simulink model "SanityCheckY"  (R2023a)
settings: Solver=VariableStepAuto  StartTime=0.0  StopTime=10.0  RelTol=1e-3
settings Model: Creator=aan18022  LastModifiedBy=aan18022

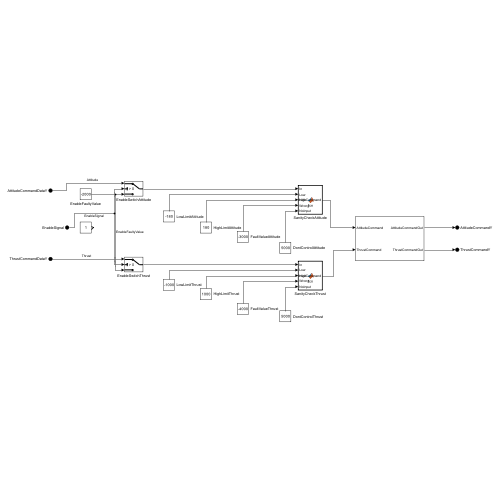
[thumbnail: Simulink's stored preview of the top-level diagram]
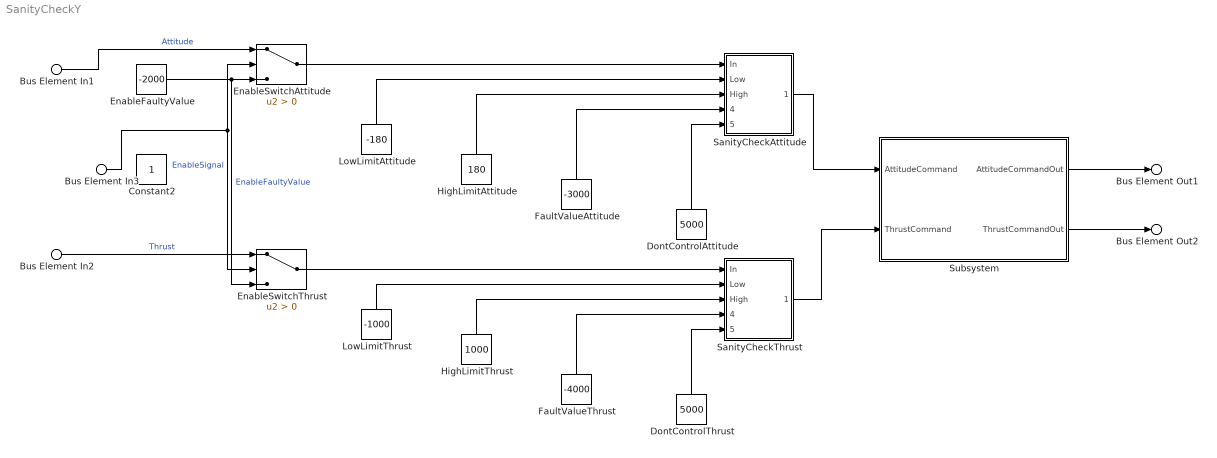
== system SanityCheckY ==
  Bus Element In3 : Inport  PortName=EnableSignal
  Bus Element In1 : Inport  Port=2  PortName=AttitudeCommandDataY
  Bus Element In2 : Inport  Port=3  PortName=ThrustCommandDataY
  Constant2 : Constant
  DontControlAttitude : Constant  Value=5000
  DontControlThrust : Constant  Value=5000
  EnableFaultyValue : Constant  Value=-2000
  EnableSwitchAttitude : Switch  Criteria=u2 > Threshold  SaturateOnIntegerOverflow=off  InputSameDT=off
  EnableSwitchThrust : Switch  Criteria=u2 > Threshold  SaturateOnIntegerOverflow=off  InputSameDT=off
  FaultValueAttitude : Constant  Value=-3000
  FaultValueThrust : Constant  Value=-4000
  HighLimitAttitude : Constant  Value=180
  HighLimitThrust : Constant  Value=1000
  LowLimitAttitude : Constant  Value=-180
  LowLimitThrust : Constant  Value=-1000
  SanityCheckAttitude : MATLAB Function  TreatAsAtomicUnit=on
  SanityCheckThrust : MATLAB Function  TreatAsAtomicUnit=on
  Subsystem : Subsystem
  Bus Element Out1 : Outport  PortName=AttitudeCommandY
  Bus Element Out2 : Outport  Port=2  PortName=ThrustCommandY
  wires:
  DontControlThrust/1 -> SanityCheckThrust/5(NoInput)
  HighLimitAttitude/1 -> SanityCheckAttitude/3(High)
  DontControlAttitude/1 -> SanityCheckAttitude/5(NoInput)
  EnableFaultyValue/1 -> EnableSwitchAttitude/3, EnableSwitchThrust/3  "EnableFaultyValue"
  Bus Element In3/1 -> EnableSwitchThrust/2, EnableSwitchAttitude/2  "EnableSignal"
  EnableSwitchThrust/1 -> SanityCheckThrust/1(In)
  FaultValueThrust/1 -> SanityCheckThrust/4(Wrong)
  HighLimitThrust/1 -> SanityCheckThrust/3(High)
  LowLimitThrust/1 -> SanityCheckThrust/2(Low)
  SanityCheckAttitude/1(AttitudeCommand) -> Subsystem/1(AttitudeCommand)
  Bus Element In2/1 -> EnableSwitchThrust/1  "Thrust"
  LowLimitAttitude/1 -> SanityCheckAttitude/2(Low)
  Bus Element In1/1 -> EnableSwitchAttitude/1  "Attitude"
  SanityCheckThrust/1(ThrustCommand) -> Subsystem/2(ThrustCommand)
  EnableSwitchAttitude/1 -> SanityCheckAttitude/1(In)
  FaultValueAttitude/1 -> SanityCheckAttitude/4(Wrong)
  Subsystem/2(ThrustCommandOut) -> Bus Element Out2/1
  Subsystem/1(AttitudeCommandOut) -> Bus Element Out1/1

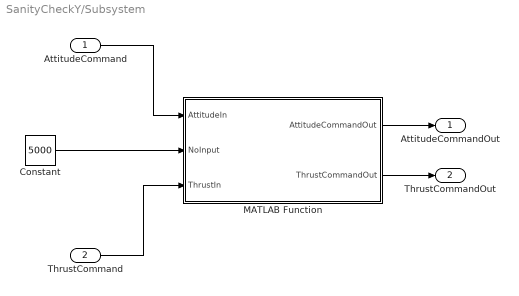
== system SanityCheckY/Subsystem ==
  AttitudeCommand : Inport
  ThrustCommand : Inport  Port=2
  Constant : Constant  Value=5000
  MATLAB Function : MATLAB Function  TreatAsAtomicUnit=on
  AttitudeCommandOut : Outport
  ThrustCommandOut : Outport  Port=2
  wires:
  AttitudeCommand/1 -> MATLAB Function/1(AttitudeIn)
  ThrustCommand/1 -> MATLAB Function/3(ThrustIn)
  MATLAB Function/1(AttitudeCommandOut) -> AttitudeCommandOut/1
  MATLAB Function/2(ThrustCommandOut) -> ThrustCommandOut/1
  Constant/1 -> MATLAB Function/2(NoInput)

== matlab function SanityCheckY/SanityCheckThrust ==
  data: In input; Out output; Low input; High input; Wrong input; NoInput input
function Out = fcn(In,Low,High,Wrong,NoInput)

if (In >=Low && In <= High)
    Out = In;
elseif In == NoInput
    Out = NoInput;
else
    Out = Wrong;
end

== matlab function SanityCheckY/SanityCheckAttitude ==
  data: In input; Out output; Low input; High input; Wrong input; NoInput input
function Out = fcn(In,Low,High,Wrong,NoInput)

if (In >=Low && In <= High)
    Out = In;
elseif In == NoInput
    Out = NoInput;
else
    Out = Wrong;
end

== matlab function SanityCheckY/Subsystem/MATLAB Function ==
  data: AttitudeIn input; NoInput input; AttitudeCommandOut output; ThrustIn input; ThrustCommandOut output
function [AttitudeCommandOut, ThrustCommandOut]= fcn(AttitudeIn, NoInput, ThrustIn)

if ThrustIn ~= NoInput
    ThrustCommandOut = ThrustIn;
    AttitudeCommandOut = NoInput;
else
    ThrustCommandOut = NoInput;
    AttitudeCommandOut = AttitudeIn;
end
